simulink model "Aalto1_ADCS_ang_vel"  (R2014a)
settings: Solver=ode3  StartTime=0.0  StopTime=6000*15  RelTol=1e-3
libraries: aausat3_lib x18, speedgoatlib_IO311 x4, slrtlib x4, xpcutilitieslib x3, dspmathops x1
settings Model: BufferReuse=off  Creator=kasperv  LastModifiedBy=Aaltosatellites
settings SolverCC: EnableConcurrentExecution=on
settings DataIOCC: SignalLoggingSaveFormat=ModelDataLogs
settings OptimizationCC: BlockReduction=off  OptimizeBlockIOStorage=off  BufferReuse=off  GlobalBufferReuse=off  ExpressionFolding=off  ExpressionDepthLimit=2147483647  LocalBlockOutputs=off
settings DebuggingCC: UnderspecifiedInitializationDetection=Classic  FcnCallInpInsideContextMsg=UseLocalSettings  StateNameClashWarn=warning
settings HardwareCC: ProdIntDivRoundTo=Zero  ProdEndianess=LittleEndian  ProdHWDeviceType=Generic->32-bit x86 compatible
settings RTWCC: SystemTargetFile=slrt.tlc  TemplateMakefile=slrt_default_tmf  Description=Simulink Real-Time  ProcessScript=slrt_make_rtw_hook  RTWCompilerOptimization=On
settings SimulinkRealTimeCC: GeneratePreprocessorConditionals=Disable all  EnableShiftOperators=on

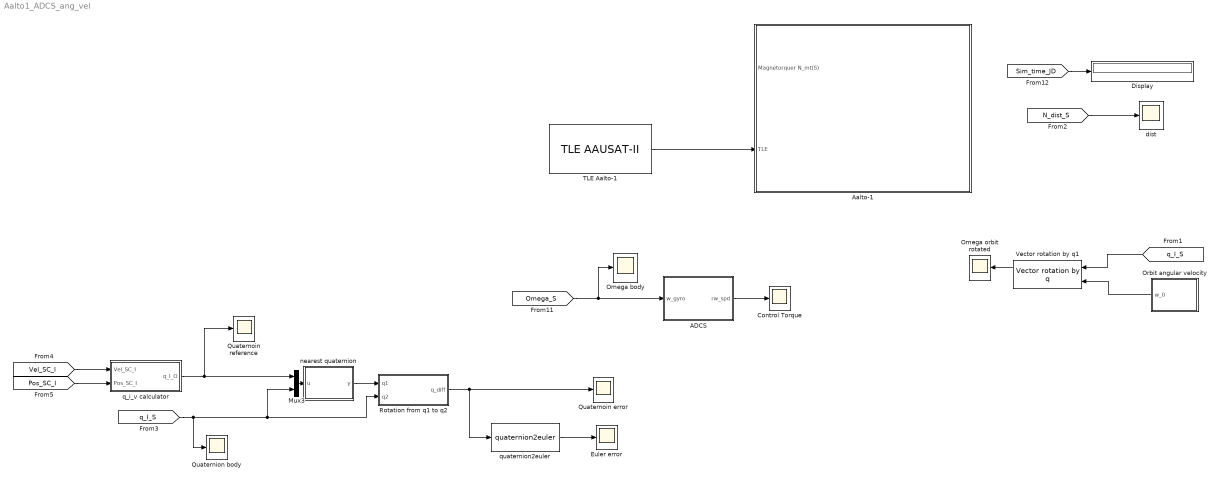
== system Aalto1_ADCS_ang_vel ==
  ADCS : Subsystem
  Aalto-1 : Subsystem  AncestorBlock=aausat3_lib/AAUSAT3  mask{r_com_s=[0.02 0.001 0.0], sat_temp_start=293.15, mass_sc=2.0, Dim=[0.207 0.1 0.1], inertia_c=[0.007,0.014,0.015], init_jd=2455153.1954318*0, q_s_c=[0 0 0 1], q_init_I_S=[0 1 0 0], w_init_s=[1,1,1]*0.2*(pi/180), Cd=2, rho=0.21850/1e12*0+9.9550/1e12*1+316.2/1e12*0, solar_m_flux=4.5565e-6, solar_absorb_coeff=1.5, theta_e=65, refldata=load('lib/AlbedoToolbox-1.0/refl_data/2005/ga050101-051231'), redfac=1, Ts=1, enable_sensor_emulation=on, enable_env_disturbance=on}
      mask prompts: r_com_s "Center of Mass:"; sat_temp_start "Start Temperature of the Satellite [K]:"; mass_sc "Mass of the Satellite [kg]:"; Dim "Satellite dimension"; inertia_c "Inertia Matrix of the Satellite:"; init_jd "Initial time [JD]:"; q_s_c "Controller Reference Frame (S->C):"; q_init_I_S "Initial Attitude (I->S):"; w_init_s "Initial Angular Rate (S) [rad/s]:"; Cd "Atmospheric Drag Coefficient [-]:"; rho "Atmospheric Density [kg/m^3]:"; solar_m_flux "Solar Momentum Flux [kg/ms^2]:"; solar_absorb_coeff "Solar Absorbtion Coefficient [-]:"; theta_e "Max. Angle of Theta [deg](eclipse: theta>r_earth/norm(R_SA)):"; refldata "Reflectivity Data (REFL Struct):"; redfac "Reduction Factor:"; Ts "Albedo Sampling Time [s]:"; enable_sensor_emulation "Enable Sensor Emulation."; enable_env_disturbance "Enable Environment Disturbance."
      mask Display:
      | image(imread('sat.jpg'));
      | color('w');
      | port_label('input', 1, 'N_mt(S)');
      | port_label('input', 2, 'TLE');
  Control Torque : Scope
      settings: TimeRange=6000  YMin=-1.1e-05  YMax=1.1e-05  SaveName=control_torque  SampleInput=on
  Display : Display
  Euler error : Scope
      settings: TimeRange=6000  YMin=-3.5  YMax=3.5  SaveName=ScopeData3  SampleInput=on
  Mux3 : Mux  Inputs=2
  Omega body : Scope
      settings: TimeRange=6000  YMin=-0.55  YMax=0.55  SaveName=ScopeData6  SampleInput=on
  Omega orbit rotated : Scope
      settings: TimeRange=6000  YMin=-0.0011  YMax=0.0011  SaveName=ScopeData9  SampleInput=on
  Orbit angular velocity : Subsystem
  Quaternion body : Scope
      settings: TimeRange=6000  YMin=-1  YMax=1  SaveName=ScopeData8  SampleInput=on
  Quaternoin error : Scope
      settings: TimeRange=7000  YMin=-0.9  YMax=1  SaveName=quaternion_error  SampleInput=on
  Quaternoin reference : Scope
      settings: TimeRange=6000  YMin=-1  YMax=1  SampleInput=on
  Rotation from q1 to q2 : Subsystem  AncestorBlock=aausat3_lib/Math Utilities/Quaternion operations/Rotation from q1 to q2
  TLE Aalto-1 : aausat3_lib/Orbit and Ephemeris/TLE AAUSAT-II  satname='Aalto-2'  JulianDay=14321.69542252  xndt2o=0.00000555  xndd6o=0.0  bstar=.76898e-4  xincl=98.6  xnodeo=12.0  eo=0.002  omegao=254.1774  xmo=105.7862  xno=14.60096319131649561528*0+15.65129795862419730331*0+16.29879739439279729389*1  ts=1
  Vector rotation by q1 : aausat3_lib/Math Utilities/Quaternion operations/Vector rotation by q
  dist : Scope
      settings: TimeRange=6000  YMin=-1e-05  YMax=1e-05  SaveName=dist  SampleInput=on
  nearest quaternion : MATLAB Function  TreatAsAtomicUnit=on
  q_i_v calculator : Subsystem
  quaternion2euler : aausat3_lib/Math Utilities/Quaternion operations/quaternion2euler
  wires:
  TLE Aalto-1/1 -> Aalto-1/2(TLE)
  [Sim_time_JD] -> Display/1
  [Pos_SC_I] -> q_i_v calculator/2(Pos_SC_I)
  [Vel_SC_I] -> q_i_v calculator/1(Vel_SC_I)
  Mux3/1 -> nearest quaternion/1(u)
  [q_I_S] -> Quaternion body/1, Rotation from q1 to q2/2(q2), Mux3/2
  quaternion2euler/1 -> Euler error/1
  q_i_v calculator/1(q_I_O) -> Mux3/1, Quaternoin reference/1
  nearest quaternion/1(y) -> Rotation from q1 to q2/1(q1)
  Vector rotation by q1/1 -> Omega orbit rotated/1
  Orbit angular velocity/1(w_0) -> Vector rotation by q1/2
  [q_I_S] -> Vector rotation by q1/1
  [N_dist_S] -> dist/1
  ADCS/1(rw_spd) -> Control Torque/1
  [Omega_S] -> ADCS/1(w_gyro), Omega body/1
  Rotation from q1 to q2/1(q_diff) -> Quaternoin error/1, quaternion2euler/1

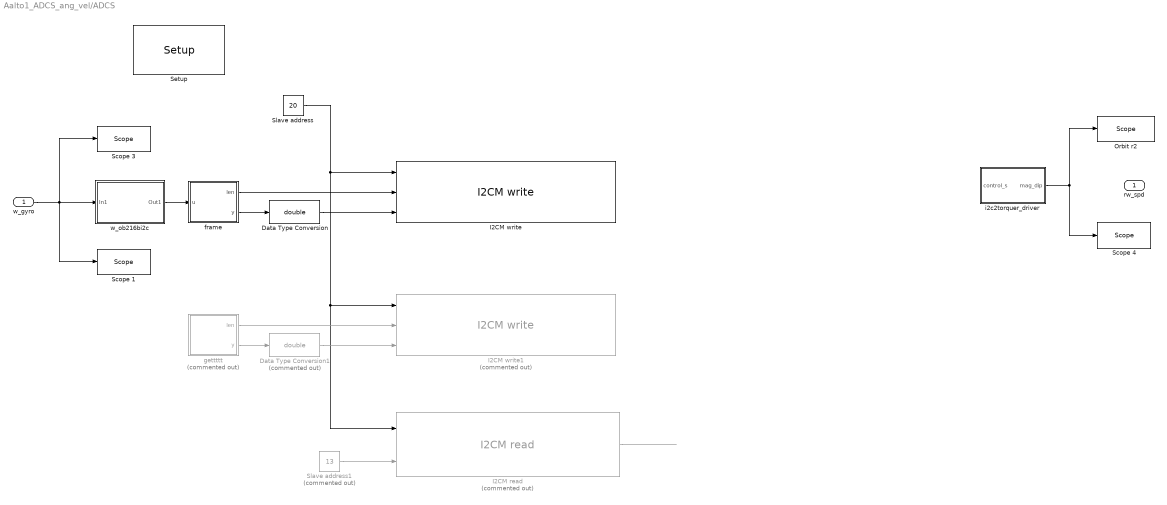
== system Aalto1_ADCS_ang_vel/ADCS ==
  w_gyro : Inport
  Data Type Conversion : DataTypeConversion  OutDataTypeStr=double
  Data Type Conversion1 : DataTypeConversion  Commented=on  OutDataTypeStr=double
  I2CM read : speedgoatlib_IO311/I2C/I2CM read  Commented=on  id=1  chan=1  clockDivider=100  subIndexConfiguration=off  ts=0.001  pciSlot=-1
  I2CM write : speedgoatlib_IO311/I2C/I2CM write  id=1  chan=1  clockDivider=100  ts=0.001  pciSlot=-1
  I2CM write1 : speedgoatlib_IO311/I2C/I2CM write  Commented=on  id=1  chan=1  clockDivider=64  ts=0.0001  pciSlot=-1
  Orbit r2 : slrtlib/Displays and Logging/Scope   scopeno=7  scopetype=File  autostart=on  viewmode=Numerical  formatstr='%15.6f'  grid=on  ylimits=[0,0]  nosamples=10000000  noprepostsamples=0  interleave=10  triggermode=Scope triggering  triggersignal=1  trigsignalfromport=off  triggerlevel=0.0  triggerslope=Either  triggerscope=1  triggersample=0  filename=dipole_m.dat  mode=Lazy  writesize=512*1024*1024  autorestart=off  dynamicfilemode=off  maxwritefilesize=512*1024^2
  Scope 1 : slrtlib/Displays and Logging/Scope   scopeno=1  scopetype=File  autostart=on  viewmode=Graphical redraw  formatstr='%15.6f'  grid=on  ylimits=[0,0]  nosamples=100000  noprepostsamples=0  interleave=1000  triggermode=FreeRun  triggersignal=1  trigsignalfromport=off  triggerlevel=0.0  triggerslope=Either  triggerscope=1  triggersample=0  filename=w_ob1.dat  mode=Lazy  writesize=512*1024  autorestart=off  dynamicfilemode=off  maxwritefilesize=512*1024^2
  Scope 3 : slrtlib/Displays and Logging/Scope   scopeno=3  scopetype=Target  autostart=on  viewmode=Graphical sliding  formatstr='%15.6f'  grid=on  ylimits=[0,0]  nosamples=1000  noprepostsamples=0  interleave=1000  triggermode=FreeRun  triggersignal=1  trigsignalfromport=off  triggerlevel=0.0  triggerslope=Either  triggerscope=1  triggersample=0  filename=w_ob1.dat  mode=Lazy  writesize=512*1024  autorestart=off  dynamicfilemode=off  maxwritefilesize=512*1024^2
  Scope 4 : slrtlib/Displays and Logging/Scope   scopeno=4  scopetype=Target  autostart=on  viewmode=Graphical sliding  formatstr='%15.6f'  grid=on  ylimits=[0,0]  nosamples=100000  noprepostsamples=0  interleave=10  triggermode=FreeRun  triggersignal=1  trigsignalfromport=off  triggerlevel=0.0  triggerslope=Either  triggerscope=1  triggersample=0  filename=w_ob1.dat  mode=Lazy  writesize=512*1024  autorestart=off  dynamicfilemode=off  maxwritefilesize=512*1024^2
  Setup : speedgoatlib_IO311/Setup/Setup  group=Lower channel group setup  id=1  fpga1=speedgoat_IO311_CI_01264  pciSlot=-1  lowerDirection=[1, 1, 0, 0, 1, 0, 1, 0, 0, 0, 0, 0, 0, 0, 0, 0]  lowerReset=[1]  lowerValue=[0]  upperDirection=[0, 0, 0, 0, 0, 0, 0, 0, 0, 0, 0, 0, 0, 0, 0, 0]  upperReset=[1]  upperValue=[0]
  Slave address : Constant  Value=20
  Slave address1 : Constant  Commented=on  Value=13
  frame : MATLAB Function  TreatAsAtomicUnit=on
  gettttt : MATLAB Function  Commented=on  TreatAsAtomicUnit=on
  i2c2torquer_driver : Subsystem
  w_ob216bi2c : Subsystem
  rw_spd : Outport
  wires:
  w_ob216bi2c/1(Out1) -> frame/1(u)
  w_gyro/1 -> Scope 1/1, Scope 3/1, w_ob216bi2c/1(In1)
  frame/2(y) -> Data Type Conversion/1
  Data Type Conversion/1 -> I2CM write/3
  i2c2torquer_driver/1(mag_dip) -> Scope 4/1, Orbit r2/1
  Slave address/1 -> I2CM read/1, I2CM write1/1, I2CM write/1
  frame/1(len) -> I2CM write/2
  Slave address1/1 -> I2CM read/2
  gettttt/2(y) -> Data Type Conversion1/1
  gettttt/1(len) -> I2CM write1/2
  Data Type Conversion1/1 -> I2CM write1/3
  I2CM read/1 -> ?

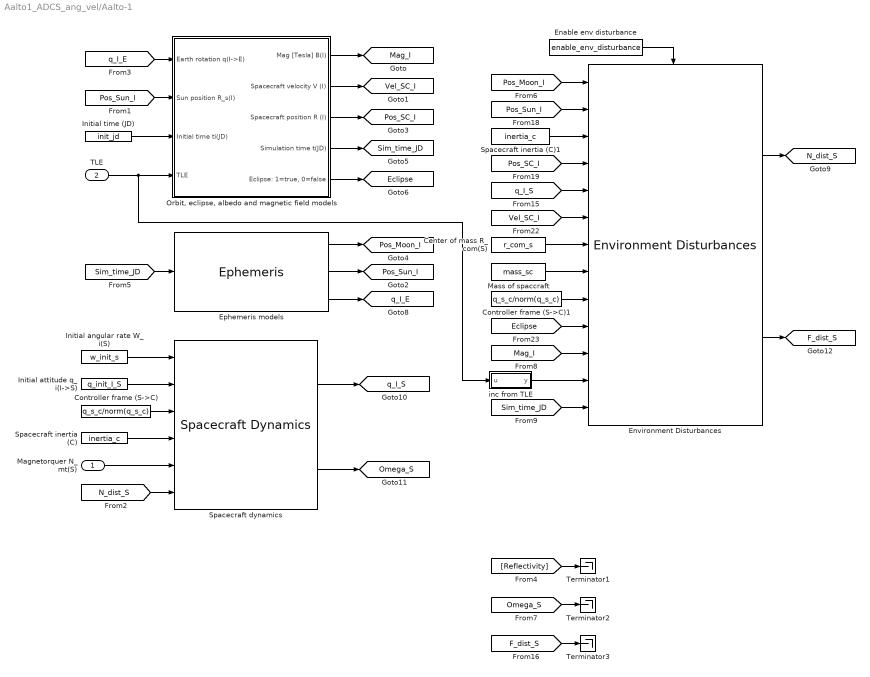
== system Aalto1_ADCS_ang_vel/Aalto-1 ==
  Magnetorquer N_mt(S) : Inport
  TLE : Inport  Port=2
  Center of mass R_com(S) : Constant  Value=r_com_s
  Controller frame (S->C) : Constant  Value=q_s_c/norm(q_s_c)
  Controller frame (S->C)1 : Constant  Value=q_s_c/norm(q_s_c)
  Enable env disturbance : Constant  Value=enable_env_disturbance
  Environment Disturbances : aausat3_lib/Disturbances/Environment Disturbances  Dim=Dim  sola_m_flux=solar_m_flux  solar_absorb_coeff=solar_absorb_coeff  rho=rho  Cd=Cd  G=6.672e-11  M_sun=1.989e30  M_earth=5.9742e24  M_moon=0.073483e24  enable_rad_dist=on  enable_atmospheric_dist=on  enable_gravity_dist=on  enable_mag_residual_dist=on
  Ephemeris models : aausat3_lib/Orbit and Ephemeris/Ephemeris
  Initial angular rate W_i(S) : Constant  Value=w_init_s
  Initial attitude q_i(I->S) : Constant  Value=q_init_I_S
  Initial time (JD) : Constant  Value=init_jd
  Mass of spaccraft : Constant  Value=mass_sc
  "Orbit, eclipse, albedo and magnetic field models" : Subsystem  AncestorBlock=aausat3_lib/Orbit and Ephemeris/Orbit and Magnetic field models  mask{theta_e=theta_e, refldata=refldata, redfac=redfac, Ts=Ts, r_e=6371e3, enable_eclipse=on, enable_IGRF=on, reflectivity_enabled=off, enable_sgp4=on, enable_custom_time=on}
      mask prompts: theta_e "Max. Angle of Theta [deg] (eclipse: theta > r_earth/norm(R_SA)):"; refldata "Reflectivity Data (REFL Struct):"; redfac "Reduction Factor:"; Ts "Albedo Model Sampling Time [s]:"; r_e "Radius of the Earth [m]:"; enable_eclipse "Enable Eclipse Model."; enable_IGRF "Enable IGRF Model."; reflectivity_enabled "Enable Albedo Model."; enable_sgp4 "Enable SGP4 Model."; enable_custom_time "Enable Custom Time."
      mask help: When you want to use "Other" make sure to define the TLE in the SGP4 subsystem.
  Spacecraft dynamics : aausat3_lib/Dynamics and Kinematics/Spacecraft Dynamics
  Spacecraft inertia (C) : Constant  Value=inertia_c
  Spacecraft inertia (C)1 : Constant  Value=inertia_c
  Terminator1 : Terminator
  Terminator2 : Terminator
  Terminator3 : Terminator
  inc from TLE : MATLAB Function  TreatAsAtomicUnit=on
  tag scope: Eclipse=global, F_dist_S=global, Mag_I=global, N_dist_S=global, Omega_S=global, Pos_Moon_I=global, Pos_SC_I=global, Pos_Sun_I=global, Sim_time_JD=global, Vel_SC_I=global, q_I_E=global, q_I_S=global
  wires:
  [q_I_S] -> Environment Disturbances/5
  Environment Disturbances/2 -> [F_dist_S]
  Environment Disturbances/1 -> [N_dist_S]
  [Mag_I] -> Environment Disturbances/11
  [Eclipse] -> Environment Disturbances/10
  Controller frame (S->C)1/1 -> Environment Disturbances/9
  Mass of spaccraft/1 -> Environment Disturbances/8
  Center of mass R_com(S)/1 -> Environment Disturbances/7
  [Vel_SC_I] -> Environment Disturbances/6
  [Pos_SC_I] -> Environment Disturbances/4
  Spacecraft inertia (C)1/1 -> Environment Disturbances/3
  [Pos_Sun_I] -> Environment Disturbances/2
  Enable env disturbance/1 -> Environment Disturbances/Enable
  [Pos_Moon_I] -> Environment Disturbances/1
  TLE/1 -> inc from TLE/1(u), "Orbit, eclipse, albedo and magnetic field models"/4(TLE)
  [q_I_E] -> "Orbit, eclipse, albedo and magnetic field models"/1(Earth rotation q(I->E))
  [Omega_S] -> Terminator2/1
  [Reflectivity] -> Terminator1/1
  Initial time (JD)/1 -> "Orbit, eclipse, albedo and magnetic field models"/3(Initial time ti(JD))
  [Pos_Sun_I] -> "Orbit, eclipse, albedo and magnetic field models"/2(Sun position R_s(I))
  Spacecraft dynamics/1 -> [q_I_S]
  [F_dist_S] -> Terminator3/1
  "Orbit, eclipse, albedo and magnetic field models"/5("Eclipse: 1=true, 0=false") -> [Eclipse]
  Magnetorquer N_mt(S)/1 -> Spacecraft dynamics/5
  "Orbit, eclipse, albedo and magnetic field models"/1(Mag [Tesla] B(I)) -> [Mag_I]
  "Orbit, eclipse, albedo and magnetic field models"/2(Spacecraft velocity V (I)) -> [Vel_SC_I]
  Spacecraft inertia (C)/1 -> Spacecraft dynamics/4
  Controller frame (S->C)/1 -> Spacecraft dynamics/3
  "Orbit, eclipse, albedo and magnetic field models"/3(Spacecraft position R (I)) -> [Pos_SC_I]
  Initial angular rate W_i(S)/1 -> Spacecraft dynamics/1
  Initial attitude q_i(I->S)/1 -> Spacecraft dynamics/2
  [Sim_time_JD] -> Environment Disturbances/13
  Ephemeris models/1 -> [Pos_Moon_I]
  Ephemeris models/2 -> [Pos_Sun_I]
  Ephemeris models/3 -> [q_I_E]
  Spacecraft dynamics/2 -> [Omega_S]
  [Sim_time_JD] -> Ephemeris models/1
  [N_dist_S] -> Spacecraft dynamics/6
  inc from TLE/1(y) -> Environment Disturbances/12
  "Orbit, eclipse, albedo and magnetic field models"/4(Simulation time t(JD)) -> [Sim_time_JD]

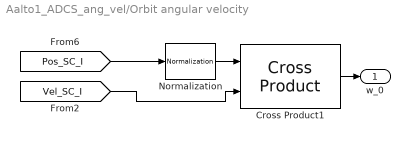
== system Aalto1_ADCS_ang_vel/Orbit angular velocity ==
  Cross Product1 : aausat3_lib/Math Utilities/Vector operations/Cross Product
  Normalization : dspmathops/Normalization  NormType=Squared 2-norm  Bias=1e-10  NormOver=Each column  ColComp=on  Dimension=1  outputDataTypeStr=Inherit: Same as product output  outputLastDataTypeStr=Inherit: Same as product output  outputMin=[]  outputMax=[]  accumDataTypeStr=Inherit: Same as product output  accumLastDataTypeStr=Inherit: Same as product output  roundingMode=Floor  overflowMode=off
  w_0 : Outport
  wires:
  Cross Product1/1 -> w_0/1
  [Vel_SC_I] -> Cross Product1/2
  [Pos_SC_I] -> Normalization/1
  Normalization/1 -> Cross Product1/1

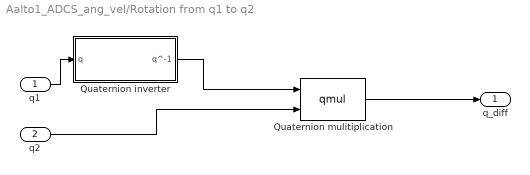
== system Aalto1_ADCS_ang_vel/Rotation from q1 to q2 ==
  q1 : Inport
  q2 : Inport  Port=2
  Quaternion inverter : Subsystem
  Quaternion mulitiplication : S-Function  FunctionName=qmul  EnableBusSupport=off
  q_diff : Outport
  wires:
  q1/1 -> Quaternion inverter/1(q)
  Quaternion inverter/1(q^-1) -> Quaternion mulitiplication/1
  q2/1 -> Quaternion mulitiplication/2
  Quaternion mulitiplication/1 -> q_diff/1

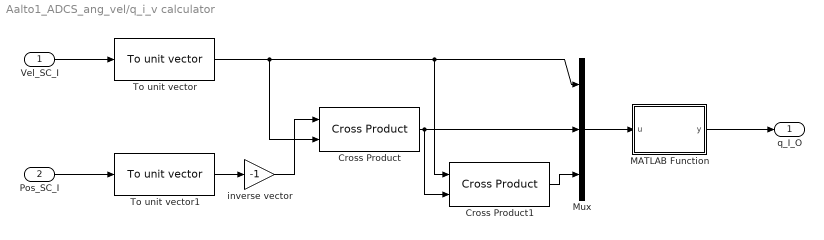
== system Aalto1_ADCS_ang_vel/q_i_v calculator ==
  Vel_SC_I : Inport
  Pos_SC_I : Inport  Port=2
  Cross Product : aausat3_lib/Math Utilities/Vector operations/Cross Product
  Cross Product1 : aausat3_lib/Math Utilities/Vector operations/Cross Product
  MATLAB Function : MATLAB Function  TreatAsAtomicUnit=on
  Mux : Mux  Inputs=3
  To unit vector : aausat3_lib/Math Utilities/Vector operations/To unit vector
  To unit vector1 : aausat3_lib/Math Utilities/Vector operations/To unit vector
  inverse vector : Gain  Gain=-1
  q_I_O : Outport
  wires:
  MATLAB Function/1(y) -> q_I_O/1
  Pos_SC_I/1 -> To unit vector1/1
  Vel_SC_I/1 -> To unit vector/1
  To unit vector/1 -> Cross Product/2, Mux/1, Cross Product1/1
  inverse vector/1 -> Cross Product/1
  To unit vector1/1 -> inverse vector/1
  Mux/1 -> MATLAB Function/1(u)
  Cross Product/1 -> Mux/2, Cross Product1/2
  Cross Product1/1 -> Mux/3

== system Aalto1_ADCS_ang_vel/ADCS/i2c2torquer_driver ==
  control_s : Inport
  Gain1 : Gain
  torquer_driver_x : Subsystem
  mag_dip : Outport
  wires:
  Gain1/1 -> mag_dip/1
  torquer_driver_x/1(Out1) -> Gain1/1
  control_s/1 -> torquer_driver_x/1(In1)

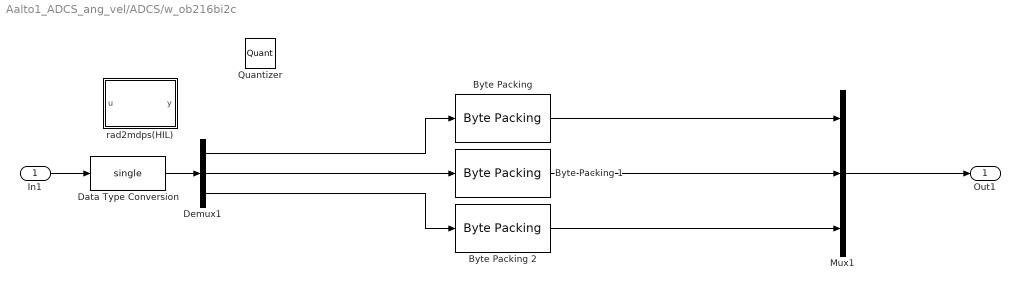
== system Aalto1_ADCS_ang_vel/ADCS/w_ob216bi2c ==
  In1 : Inport
  "Byte Packing " : xpcutilitieslib/Byte Packing   MaskPackedDataType=uint8  MaskUnpackedDataTypes={'single'}  MaskAlignment=1
  Byte Packing 1 : xpcutilitieslib/Byte Packing   MaskPackedDataType=uint8  MaskUnpackedDataTypes={'single'}  MaskAlignment=1
  Byte Packing 2 : xpcutilitieslib/Byte Packing   MaskPackedDataType=uint8  MaskUnpackedDataTypes={'single'}  MaskAlignment=1
  Data Type Conversion : DataTypeConversion  OutDataTypeStr=single
  Demux1 : Demux  Outputs=3
  Mux1 : Mux  Inputs=3
  Quantizer : Quantizer  QuantizationInterval=1
  rad2mdps(HIL) : MATLAB Function  TreatAsAtomicUnit=on
  Out1 : Outport
  wires:
  Mux1/1 -> Out1/1
  ? -> Quantizer/1
  Demux1/2 -> Byte Packing 1/1
  In1/1 -> Data Type Conversion/1
  Demux1/1 -> "Byte Packing "/1
  Demux1/3 -> Byte Packing 2/1
  Data Type Conversion/1 -> Demux1/1
  Byte Packing 2/1 -> Mux1/3
  Byte Packing 1/1 -> Mux1/2
  "Byte Packing "/1 -> Mux1/1

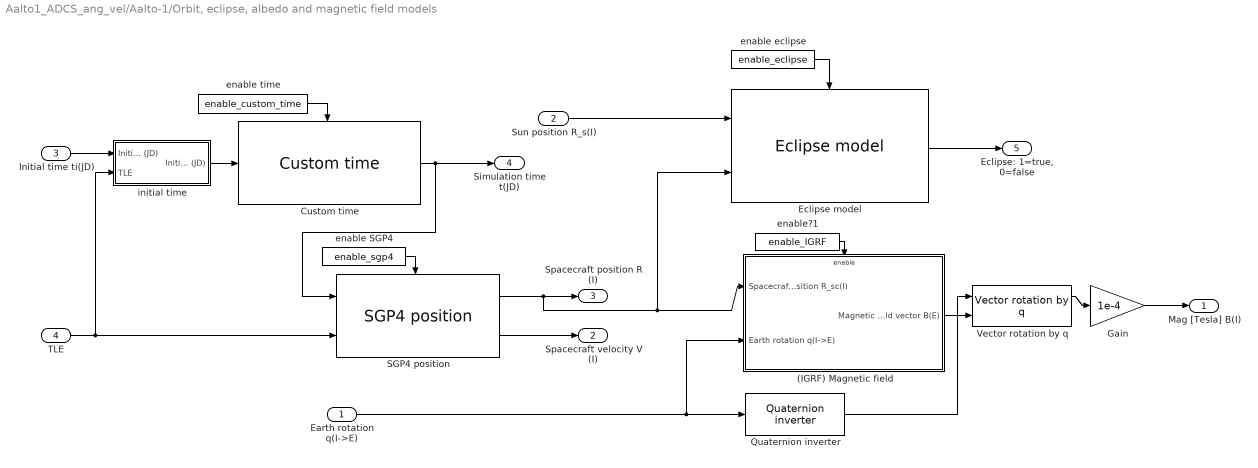
== system Aalto1_ADCS_ang_vel/Aalto-1/Orbit, eclipse, albedo and magnetic field models ==
  Earth rotation q(I->E) : Inport
  Sun position R_s(I) : Inport  Port=2
  Initial time ti(JD) : Inport  Port=3
  TLE : Inport  Port=4
  (IGRF) Magnetic field : Subsystem  AncestorBlock=aausat3_lib/Orbit and Ephemeris/(IGRF) Magnetic field  TreatAsAtomicUnit=on
  Custom time : aausat3_lib/Orbit and Ephemeris/Custom time
  Eclipse model : aausat3_lib/Orbit and Ephemeris/Eclipse model  r_e=r_e  enable=off  theta_e=theta_e
  Gain : Gain  Gain=1e-4
  Quaternion inverter : aausat3_lib/Math Utilities/Quaternion operations/Quaternion inverter
  SGP4 position : aausat3_lib/Orbit and Ephemeris/SGP4 position
  Vector rotation by q : aausat3_lib/Math Utilities/Quaternion operations/Vector rotation by q
  enable SGP4 : Constant  Value=enable_sgp4
  enable eclipse : Constant  Value=enable_eclipse
  enable time : Constant  Value=enable_custom_time
  enable?1 : Constant  Value=enable_IGRF
  initial time : Subsystem
  Mag [Tesla] B(I) : Outport
  Spacecraft velocity V (I) : Outport  Port=2
  Spacecraft position R (I) : Outport  Port=3
  Simulation time t(JD) : Outport  Port=4
  "Eclipse: 1=true, 0=false" : Outport  Port=5  PortDimensions=1
  wires:
  Initial time ti(JD)/1 -> initial time/1(Initial time in (JD))
  initial time/1(Initial time out (JD)) -> Custom time/1
  TLE/1 -> initial time/2(TLE), SGP4 position/2
  enable eclipse/1 -> Eclipse model/Enable
  Gain/1 -> Mag [Tesla] B(I)/1
  (IGRF) Magnetic field/1(Magnetic field vector B(E)) -> Vector rotation by q/2
  SGP4 position/2 -> Spacecraft velocity V (I)/1
  SGP4 position/1 -> Spacecraft position R (I)/1, Eclipse model/2, (IGRF) Magnetic field/1(Spacecraft position R_sc(I))
  enable SGP4/1 -> SGP4 position/Enable
  Earth rotation q(I->E)/1 -> Quaternion inverter/1, (IGRF) Magnetic field/2(Earth rotation q(I->E))
  Sun position R_s(I)/1 -> Eclipse model/1
  Custom time/1 -> SGP4 position/1, Simulation time t(JD)/1
  enable time/1 -> Custom time/Enable
  Quaternion inverter/1 -> Vector rotation by q/1
  Vector rotation by q/1 -> Gain/1
  enable?1/1 -> (IGRF) Magnetic field/Enable
  Eclipse model/1 -> "Eclipse: 1=true, 0=false"/1

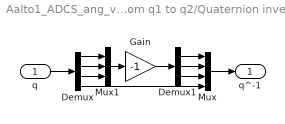
== system Aalto1_ADCS_ang_vel/Rotation from q1 to q2/Quaternion inverter ==
  q : Inport
  Demux : Demux
  Demux1 : Demux  Outputs=3
  Gain : Gain  Gain=-1  SaturateOnIntegerOverflow=on  OutDataTypeStr=Inherit: Same as input  ParamDataTypeStr=Inherit: Same as input
  Mux : Mux
  Mux1 : Mux  Inputs=3
  q^-1 : Outport
  wires:
  q/1 -> Demux/1
  Mux/1 -> q^-1/1
  Demux/4 -> Mux/4
  Demux/1 -> Mux1/1
  Demux/2 -> Mux1/2
  Demux/3 -> Mux1/3
  Mux1/1 -> Gain/1
  Demux1/1 -> Mux/1
  Demux1/2 -> Mux/2
  Demux1/3 -> Mux/3
  Gain/1 -> Demux1/1

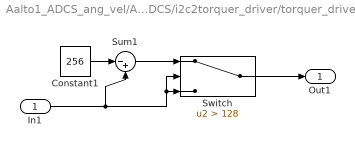
== system Aalto1_ADCS_ang_vel/ADCS/i2c2torquer_driver/torquer_driver_x ==
  In1 : Inport
  Constant1 : Constant  Value=256
  Sum1 : Sum  Inputs=|-+
  Switch : Switch  Criteria=u2 > Threshold  Threshold=128
  Out1 : Outport
  wires:
  In1/1 -> Sum1/2, Switch/2, Switch/3
  Constant1/1 -> Sum1/1
  Sum1/1 -> Switch/1
  Switch/1 -> Out1/1

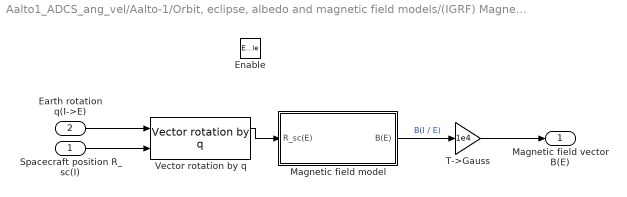
== system Aalto1_ADCS_ang_vel/Aalto-1/Orbit, eclipse, albedo and magnetic field models/(IGRF) Magnetic field ==
  Spacecraft position R_sc(I) : Inport
  Earth rotation q(I->E) : Inport  Port=2
  Enable : EnablePort
  Magnetic field model : Subsystem
  T->Gauss : Gain  Gain=1e4  SaturateOnIntegerOverflow=on  OutDataTypeStr=Inherit: Same as input  ParamDataTypeStr=Inherit: Same as input
  Vector rotation by q : aausat3_lib/Math Utilities/Quaternion operations/Vector rotation by q
  Magnetic field vector B(E) : Outport
  wires:
  Spacecraft position R_sc(I)/1 -> Vector rotation by q/2
  Earth rotation q(I->E)/1 -> Vector rotation by q/1
  Vector rotation by q/1 -> Magnetic field model/1(R_sc(E))
  Magnetic field model/1(B(E)) -> T->Gauss/1  "B(I / E)"
  T->Gauss/1 -> Magnetic field vector B(E)/1

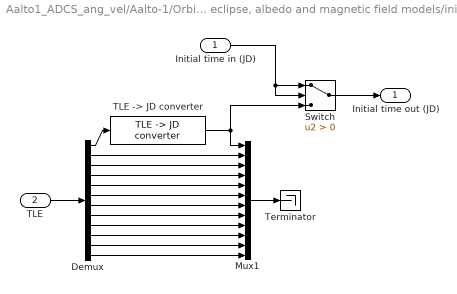
== system Aalto1_ADCS_ang_vel/Aalto-1/Orbit, eclipse, albedo and magnetic field models/initial time ==
  Initial time in (JD) : Inport
  TLE : Inport  Port=2
  Demux : Demux  Outputs=12
  Mux1 : Mux  Inputs=12
  Switch : Switch  Criteria=u2 > Threshold
  "TLE -> JD converter" : aausat3_lib/Other Model Utilities/TLE -> JD converter
  Terminator : Terminator
  Initial time out (JD) : Outport
  wires:
  Mux1/1 -> Terminator/1
  Switch/1 -> Initial time out (JD)/1
  Initial time in (JD)/1 -> Switch/1, Switch/2
  TLE/1 -> Demux/1
  Demux/2 -> Mux1/2
  Demux/3 -> Mux1/3
  Demux/4 -> Mux1/4
  Demux/5 -> Mux1/5
  Demux/6 -> Mux1/6
  Demux/7 -> Mux1/7
  Demux/8 -> Mux1/8
  Demux/9 -> Mux1/9
  Demux/10 -> Mux1/10
  Demux/11 -> Mux1/11
  Demux/12 -> Mux1/12
  Demux/1 -> "TLE -> JD converter"/1
  "TLE -> JD converter"/1 -> Switch/3, Mux1/1

== system Aalto1_ADCS_ang_vel/Aalto-1/Orbit, eclipse, albedo and magnetic field models/(IGRF) Magnetic field/Magnetic field model ==
  R_sc(E) : Inport
  S-Function : S-Function  FunctionName=igrfS2  Parameters=2009,13  EnableBusSupport=off
  B(E) : Outport
  wires:
  S-Function/1 -> B(E)/1
  R_sc(E)/1 -> S-Function/1

== matlab function Aalto1_ADCS_ang_vel/nearest quaternion ==
  data: u input; y output
function y = fcn(u)
     q = u(1:4);
     p = u(5:8);
     y = [q_pick_near(p', q')']; 
     
end

== matlab function Aalto1_ADCS_ang_vel/ADCS/w_ob216bi2c/rad2mdps(HIL) ==
  data: u input; y output
function y = fcn(u)
%#codegen

flag = u < 0;
y = (2^32+1.*flag + u)*180/pi*1000;

== matlab function Aalto1_ADCS_ang_vel/q_i_v calculator/MATLAB Function ==
  data: u input; y output
function y = fcn(u)
%#codegen

y = dcmatrix_and_q(u);

== matlab function Aalto1_ADCS_ang_vel/ADCS/frame ==
  data: len output; u input; y output uint8
function [len,y] = fcn(u)
%#codegen
u
y = [170; 177; 14; fliplr(u(1:4)')'; fliplr(u(5:8)')'; fliplr(u(9:12)')'; zeros(49, 1)];
y(4:15)
%y = [170; 177; 14; u; zeros(49, 1)];

len = 12; % size(y,1)

== matlab function Aalto1_ADCS_ang_vel/ADCS/gettttt ==
  data: len output; y output uint8
function [len,y] = fcn()
%#codegen

y = [170; 180; 0; 0];

len = 4; % size(y,1)

== matlab function Aalto1_ADCS_ang_vel/Aalto-1/inc from TLE ==
  data: u input; y output
function y = fcn(u)
%#codegen

y = u(7);
